simulink model "ex_13_7_dsb"  (R2021b)
settings: Solver=ode45  StartTime=0.0  StopTime=10  RelTol=1e-3  EnableMultiTasking=on
libraries: commanapbnd3 x2
settings Model: Creator=Yuantao  LastModifiedBy=Yuantao
settings SolverCC: AlgebraicLoopSolver=TrustRegion
settings DataIOCC: LimitDataPoints=on  SaveFormat=Array  SignalLoggingSaveFormat=ModelDataLogs  ReturnWorkspaceOutputs=off
settings OptimizationCC: InitFltsAndDblsToZero=on  LifeSpan=inf
settings DebuggingCC: SaveWithParameterizedLinksMsg=none  UnderspecifiedInitializationDetection=Classic  MergeDetectMultiDrivingBlocksExec=none  SignalResolutionControl=TryResolveAllWithWarning  SolverPrmCheckMsg=warning  MultiTaskDSMMsg=warning  MultiTaskCondExecSysMsg=none  FcnCallInpInsideContextMsg=warning  SFUnexpectedBacktrackingDiag=warning  SFNoUnconditionalDefaultTransitionDiag=warning  SFExecutionAtInitializationDiag=none  SFMachineParentedDataDiag=warning  ArithmeticOperatorsInVariantConditions=warning
settings HardwareCC: ProdBitPerPointer=32  ProdBitPerSizeT=32  ProdBitPerPtrDiffT=32  ProdLargestAtomicFloat=None  ProdIntDivRoundTo=Undefined  ProdEndianess=Unspecified  ProdWordSize=32  ProdHWDeviceType=32-bit Generic
settings ModelReferenceCC: PropagateSignalLabelsOutOfModel=off
settings CodeAppCC: StateflowObjectComments=on
settings GRTTargetCC: TargetFcnLib=ansi_tfl_tmw.mat  TargetLangStandard=C89/C90 (ANSI)  CombineOutputUpdateFcns=off  GRTInterface=on
settings ConfigComp: CovMetricSettings=dw  CovSaveCumulativeToWorkspaceVar=on  CovSaveSingleToWorkspaceVar=on

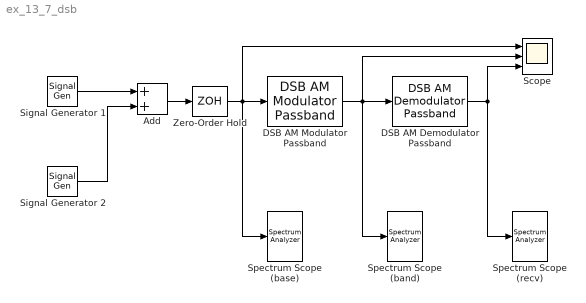
== system ex_13_7_dsb ==
  Add : Sum
  DSB AM Demodulator Passband : commanapbnd3/DSB AM Demodulator Passband  Fc=100  Ph=0  method=Butterworth  n=4  cf=30  Rp=1  Rs=1  Offset=0
      settings: SourceProductBaseCode=CM
  DSB AM Modulator Passband : commanapbnd3/DSB AM Modulator Passband  Fc=100  Ph=0  Offset=0
      settings: SourceProductBaseCode=CM
  Scope : Scope  NumInputPorts=3
      settings: AttributesFormatString='r'=%<ForegroundColor>
  Signal Generator 1 : SignalGenerator  Amplitude=3  Frequency=10
  Signal Generator 2 : SignalGenerator  Amplitude=2  Frequency=20
  Spectrum Scope (band) : SpectrumAnalyzer
  Spectrum Scope (base) : SpectrumAnalyzer
  Spectrum Scope (recv) : SpectrumAnalyzer
  Zero-Order Hold : ZeroOrderHold  SampleTime=0.002
  wires:
  Signal Generator 1/1 -> Add/1
  DSB AM Modulator Passband/1 -> Spectrum Scope (band)/1, DSB AM Demodulator Passband/1, Scope/2
  DSB AM Demodulator Passband/1 -> Spectrum Scope (recv)/1, Scope/3
  Add/1 -> Zero-Order Hold/1
  Signal Generator 2/1 -> Add/2
  Zero-Order Hold/1 -> Spectrum Scope (base)/1, DSB AM Modulator Passband/1, Scope/1
